simulink model "sat_orbit_orientation_propSIM_tmp"  (R2019b)
settings: Solver=ode45  StartTime=0.0  StopTime=15000.0  MaxStep=0.009  RelTol=1e-6
libraries: simulink x2
settings Model: Creator=Hector  LastModifiedBy=Hector
settings SolverCC: AlgebraicLoopSolver=LineSearch

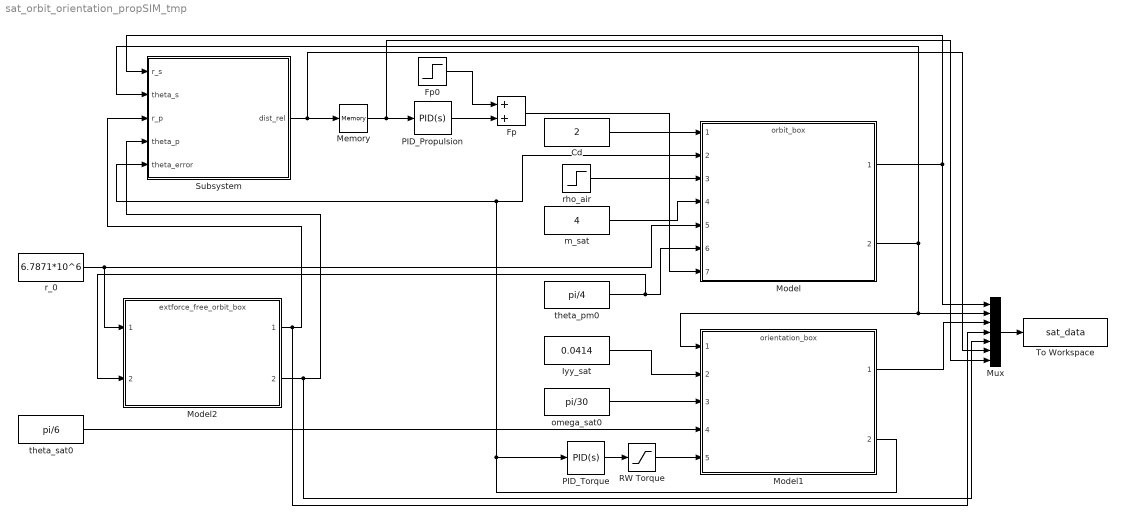
== system sat_orbit_orientation_propSIM_tmp ==
  Cd : Constant  Value=2
  Fp : Sum
  Fp0 : Step  Time=0  After=1.28835626946219*10^(-6)  SampleTime=0
  Iyy_sat : Constant  Value=0.0414
  Memory : Memory
  Model : ModelReference  ModelNameDialog=orbit_box.slx  SimulationMode=Normal  ModelReferenceVersion=1.34
  Model1 : ModelReference  ModelNameDialog=orientation_box.slx  SimulationMode=Normal  ModelReferenceVersion=1.29
  Model2 : ModelReference  ModelNameDialog=extforce_free_orbit_box.slx  SimulationMode=Normal  ModelReferenceVersion=1.34
  Mux : Mux  Inputs=7
  PID_Propulsion : simulink/Continuous/PID Controller  Controller=PID  Form=Parallel  TimeDomain=Continuous-time  SampleTime=-1  IntegratorMethod=Forward Euler  FilterMethod=Forward Euler  ControllerParametersSource=internal  P=2.11519715784155e-06  I=1.28628982869464e-10  D=0.00754921104528398  UseFilter=on  N=0.228565595208321  TunerSelectOption=Transfer Function Based (PID Tuner App)  InitialConditionSource=internal  InitialConditionForIntegrator=0  InitialConditionForFilter=0  DifferentiatorICPrevScaledInput=0  ExternalReset=none  TrackingMode=off  Kt=1  LimitOutput=off  UpperSaturationLimit=.05e-03  LowerSaturationLimit=0  LinearizeAsGain=off  AntiWindupMode=none  Kb=1  POutMin=[]  POutMax=[]  IOutMin=[]  IOutMax=[]  DOutMin=[]  DOutMax=[]  NOutMin=[]  NOutMax=[]  SumOutMin=[]  SumOutMax=[]  SaturationOutMin=[]  SaturationOutMax=[]  PParamMin=[]  PParamMax=[]  IParamMin=[]  IParamMax=[]  DParamMin=[]  DParamMax=[]  NParamMin=[]  NParamMax=[]  KbParamMin=[]  KbParamMax=[]  KtParamMin=[]  KtParamMax=[]  KbOutMin=[]  KbOutMax=[]  KtOutMin=[]  KtOutMax=[]  IntegratorOutMin=[]  IntegratorOutMax=[]  FilterOutMin=[]  FilterOutMax=[]  SumI1OutMin=[]  SumI1OutMax=[]  SumI2OutMin=[]  SumI2OutMax=[]  SumI3OutMin=[]  SumI3OutMax=[]  SumI4OutMin=[]  SumI4OutMax=[]  SumDOutMin=[]  SumDOutMax=[]  DifferentiatorOutMin=[]  DifferentiatorOutMax=[]  FilterDiffOutCoefMin=[]  FilterDiffOutCoefMax=[]  ReciprocalOutMin=[]  ReciprocalOutMax=[]  SumDenOutMin=[]  SumDenOutMax=[]  SumNumOutMin=[]  SumNumOutMax=[]  DivideOutMin=[]  DivideOutMax=[]  IntegratorContinuousStateAttributes=''  IntegratorStateMustResolveToSignalObject=off  IntegratorRTWStateStorageClass=Auto  FilterContinuousStateAttributes=''  FilterStateMustResolveToSignalObject=off  FilterRTWStateStorageClass=Auto  ParallelPVariant=InternalParameters  IdealPVariant=Disabled  IVariant=InternalParameters  DVariant=InternalParameters  IntegratorVariant=Continuous  SatVariant=Disabled  AWVariant=Passthrough  PCopyVariant=Disabled  TRVariant=Disabled  FdbkBlocksVariant=Forward  IdealPFdbkVariant=Disabled  SatFdbkVariant=Disabled  DerivativeFilterVariant=ContFilter  NVariant=InternalParameters  NCopyVariant=Disabled  FilterICVariant=InternalICsFilter  IntegratorICVariant=InternalICs  ExternalResetVariant=Disabled  TRSumVariant=Passthrough  SumFdbkVariant=Disabled  SumVariant=Sum_PID
  PID_Torque : simulink/Continuous/PID Controller  Controller=PID  Form=Parallel  TimeDomain=Continuous-time  SampleTime=-1  IntegratorMethod=Forward Euler  FilterMethod=Forward Euler  ControllerParametersSource=internal  P=5.33827881904527e-05  I=2.08258616091013e-07  D=0.00336002738651377  UseFilter=on  N=0.454497521184683  TunerSelectOption=Transfer Function Based (PID Tuner App)  InitialConditionSource=internal  InitialConditionForIntegrator=0  InitialConditionForFilter=0  DifferentiatorICPrevScaledInput=0  ExternalReset=none  TrackingMode=off  Kt=1  LimitOutput=off  UpperSaturationLimit=inf  LowerSaturationLimit=-inf  LinearizeAsGain=on  AntiWindupMode=none  Kb=1  POutMin=[]  POutMax=[]  IOutMin=[]  IOutMax=[]  DOutMin=[]  DOutMax=[]  NOutMin=[]  NOutMax=[]  SumOutMin=[]  SumOutMax=[]  SaturationOutMin=[]  SaturationOutMax=[]  PParamMin=[]  PParamMax=[]  IParamMin=[]  IParamMax=[]  DParamMin=[]  DParamMax=[]  NParamMin=[]  NParamMax=[]  KbParamMin=[]  KbParamMax=[]  KtParamMin=[]  KtParamMax=[]  KbOutMin=[]  KbOutMax=[]  KtOutMin=[]  KtOutMax=[]  IntegratorOutMin=[]  IntegratorOutMax=[]  FilterOutMin=[]  FilterOutMax=[]  SumI1OutMin=[]  SumI1OutMax=[]  SumI2OutMin=[]  SumI2OutMax=[]  SumI3OutMin=[]  SumI3OutMax=[]  SumI4OutMin=[]  SumI4OutMax=[]  SumDOutMin=[]  SumDOutMax=[]  DifferentiatorOutMin=[]  DifferentiatorOutMax=[]  FilterDiffOutCoefMin=[]  FilterDiffOutCoefMax=[]  ReciprocalOutMin=[]  ReciprocalOutMax=[]  SumDenOutMin=[]  SumDenOutMax=[]  SumNumOutMin=[]  SumNumOutMax=[]  DivideOutMin=[]  DivideOutMax=[]  IntegratorContinuousStateAttributes=''  IntegratorStateMustResolveToSignalObject=off  IntegratorRTWStateStorageClass=Auto  FilterContinuousStateAttributes=''  FilterStateMustResolveToSignalObject=off  FilterRTWStateStorageClass=Auto  ParallelPVariant=InternalParameters  IdealPVariant=Disabled  IVariant=InternalParameters  DVariant=InternalParameters  IntegratorVariant=Continuous  SatVariant=Disabled  AWVariant=Passthrough  PCopyVariant=Disabled  TRVariant=Disabled  FdbkBlocksVariant=Forward  IdealPFdbkVariant=Disabled  SatFdbkVariant=Disabled  DerivativeFilterVariant=ContFilter  NVariant=InternalParameters  NCopyVariant=Disabled  FilterICVariant=InternalICsFilter  IntegratorICVariant=InternalICs  ExternalResetVariant=Disabled  TRSumVariant=Passthrough  SumFdbkVariant=Disabled  SumVariant=Sum_PID
  RW Torque : Saturate  UpperLimit=0.00023  LowerLimit=-0.00023
  Subsystem : Subsystem
  To Workspace : ToWorkspace  VariableName=sat_data  SampleTime=-1
  m_sat : Constant  Value=4
  omega_sat0 : Constant  Value=pi/30
  r_0 : Constant  Value=6.7871*10^6
  rho_air : Step  Time=0  After=0.219*10^(-11)  SampleTime=0
  theta_pm0 : Constant  Value=pi/4
  theta_sat0 : Constant  Value=pi/6
  wires:
  Cd/1 -> Model/1
  Model1/2 -> PID_Torque/1, Model/2, Subsystem/5(theta_error)
  rho_air/1 -> Model/3
  m_sat/1 -> Model/4
  r_0/1 -> Model/5, Model2/1
  theta_pm0/1 -> Model2/2, Model/6
  Model/2 -> Mux/2, Model1/1, Subsystem/2(theta_s)
  Iyy_sat/1 -> Model1/2
  omega_sat0/1 -> Model1/3
  theta_sat0/1 -> Model1/4
  PID_Torque/1 -> RW Torque/1
  RW Torque/1 -> Model1/5
  Model/1 -> Mux/1, Subsystem/1(r_s)
  Mux/1 -> To Workspace/1
  Model1/1 -> Mux/3
  Model2/1 -> Mux/4, Subsystem/3(r_p)
  Model2/2 -> Mux/5, Subsystem/4(theta_p)
  Fp0/1 -> Fp/1
  PID_Propulsion/1 -> Fp/2
  Fp/1 -> Model/7
  Memory/1 -> Mux/7, PID_Propulsion/1
  Subsystem/1(dist_rel) -> Memory/1, Mux/6

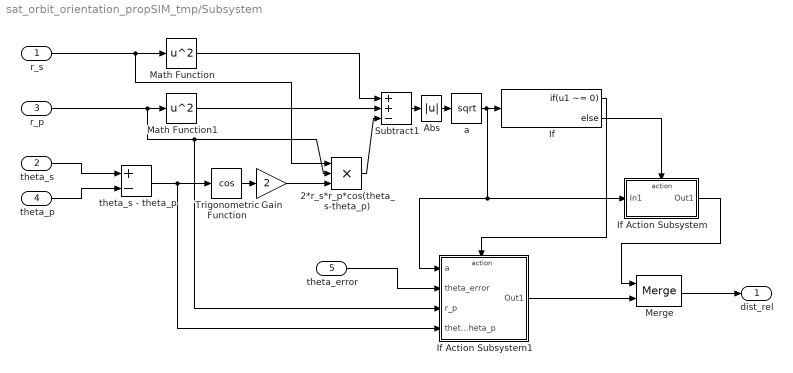
== system sat_orbit_orientation_propSIM_tmp/Subsystem ==
  r_s : Inport
  theta_s : Inport  Port=2
  r_p : Inport  Port=3
  theta_p : Inport  Port=4
  theta_error : Inport  Port=5
  2*r_s*r_p*cos(theta_s-theta_p) : Product  Inputs=3
  Abs : Abs
  Gain : Gain  Gain=2
  If : If  IfExpression=u1 ~= 0
  If Action Subsystem : Subsystem  TreatAsAtomicUnit=on
  If Action Subsystem1 : Subsystem  TreatAsAtomicUnit=on
  Math Function : Math  Operator=square  SignedPower=off  SaturateOnIntegerOverflow=on
  Math Function1 : Math  Operator=square  SignedPower=off  SaturateOnIntegerOverflow=on
  Merge : Merge
  Subtract1 : Sum  Inputs=++-
  Trigonometric Function : Trigonometry  Operator=cos
  a : Sqrt  SaturateOnIntegerOverflow=on
  theta_s - theta_p : Sum  Inputs=+-
  dist_rel : Outport
  wires:
  r_p/1 -> If Action Subsystem1/3(r_p), 2*r_s*r_p*cos(theta_s-theta_p)/2, Math Function1/1
  theta_s/1 -> theta_s - theta_p/1
  theta_p/1 -> theta_s - theta_p/2
  theta_s - theta_p/1 -> If Action Subsystem1/4(theta_s - theta_p), Trigonometric Function/1
  r_s/1 -> Math Function/1, 2*r_s*r_p*cos(theta_s-theta_p)/1
  Trigonometric Function/1 -> Gain/1
  Gain/1 -> 2*r_s*r_p*cos(theta_s-theta_p)/3
  Math Function/1 -> Subtract1/1
  Math Function1/1 -> Subtract1/2
  2*r_s*r_p*cos(theta_s-theta_p)/1 -> Subtract1/3
  a/1 -> If Action Subsystem1/1(a), If Action Subsystem/1(In1), If/1
  If/1 -> If Action Subsystem1/Action
  If/2 -> If Action Subsystem/Action
  theta_error/1 -> If Action Subsystem1/2(theta_error)
  If Action Subsystem/1(Out1) -> Merge/1
  If Action Subsystem1/1(Out1) -> Merge/2
  Merge/1 -> dist_rel/1
  Subtract1/1 -> Abs/1
  Abs/1 -> a/1

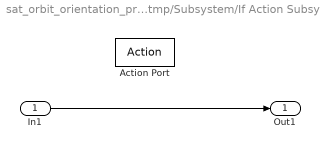
== system sat_orbit_orientation_propSIM_tmp/Subsystem/If Action Subsystem ==
  In1 : Inport
  Action Port : ActionPort  ActionPortLabel=else
  Out1 : Outport
  wires:
  In1/1 -> Out1/1

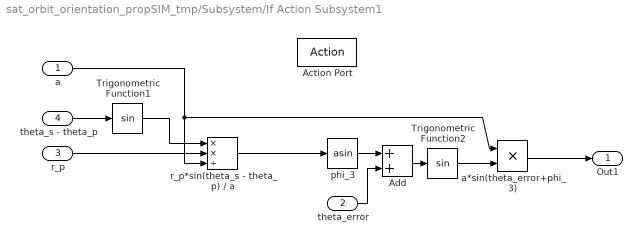
== system sat_orbit_orientation_propSIM_tmp/Subsystem/If Action Subsystem1 ==
  a : Inport
  theta_error : Inport  Port=2
  r_p : Inport  Port=3
  theta_s - theta_p : Inport  Port=4
  Action Port : ActionPort  ActionPortLabel=if(u1 ~= 0)
  Add : Sum
  Trigonometric Function1 : Trigonometry
  Trigonometric Function2 : Trigonometry
  a*sin(theta_error+phi_3) : Product
  phi_3 : Trigonometry  Operator=asin
  r_p*sin(theta_s - theta_p) / a : Product  Inputs=**/
  Out1 : Outport
  wires:
  theta_error/1 -> Add/2
  a/1 -> a*sin(theta_error+phi_3)/1, r_p*sin(theta_s - theta_p) / a/3
  Add/1 -> Trigonometric Function2/1
  r_p*sin(theta_s - theta_p) / a/1 -> phi_3/1
  r_p/1 -> r_p*sin(theta_s - theta_p) / a/2
  phi_3/1 -> Add/1
  Trigonometric Function2/1 -> a*sin(theta_error+phi_3)/2
  Trigonometric Function1/1 -> r_p*sin(theta_s - theta_p) / a/1
  theta_s - theta_p/1 -> Trigonometric Function1/1
  a*sin(theta_error+phi_3)/1 -> Out1/1
